simulink model "ClosedLoop"  (R2018b)
(part 3 of 12)

  "IW{1,1}(79,:)'" : Constant  Value=[0.15874800000000000022026824808563105762004852294921875;-0.25384499999999998731681216668221168220043182373046875;-0.29713800000000001322320031249546445906162261962890625]
      mask Display: e = 0.06;c1 = [120 150 230]/255;c2 = ([120 150 230]+0)/383;c3 = ([120 150 230]+128)/383;patch([0 1 1 0],[0 0 1 1],c1);patch([0 1 1 1-e 1-e 0+e],[0 0 1 1-e 0+e 0+e],c2);patch([0 0 1 1-e 0+e 0+e],[0 1 1 1-e 1-e 0+e],c3);plot([0 1 1 0 0],[0 0 1 1 0]);disp('Weights');
  "IW{1,1}(8,:)'" : Constant  Value=[-1.2600000000000000088817841970012523233890533447265625;-1.2874399999999999177902054725564084947109222412109375;0.01036259999999999958930629873066209256649017333984375]
      mask Display: e = 0.06;c1 = [120 150 230]/255;c2 = ([120 150 230]+0)/383;c3 = ([120 150 230]+128)/383;patch([0 1 1 0],[0 0 1 1],c1);patch([0 1 1 1-e 1-e 0+e],[0 0 1 1-e 0+e 0+e],c2);patch([0 0 1 1-e 0+e 0+e],[0 1 1 1-e 1-e 0+e],c3);plot([0 1 1 0 0],[0 0 1 1 0]);disp('Weights');
  "IW{1,1}(80,:)'" : Constant  Value=[0.048155099999999999293986974180370452813804149627685546875;0.0320770999999999972818187643497367389500141143798828125;-0.045470900000000001595079623939454904757440090179443359375]
      mask Display: e = 0.06;c1 = [120 150 230]/255;c2 = ([120 150 230]+0)/383;c3 = ([120 150 230]+128)/383;patch([0 1 1 0],[0 0 1 1],c1);patch([0 1 1 1-e 1-e 0+e],[0 0 1 1-e 0+e 0+e],c2);patch([0 0 1 1-e 0+e 0+e],[0 1 1 1-e 1-e 0+e],c3);plot([0 1 1 0 0],[0 0 1 1 0]);disp('Weights');
  "IW{1,1}(81,:)'" : Constant  Value=[0.007354610000000000140374378787555542658083140850067138671875;-0.0310646000000000012397638471384198055602610111236572265625;0.0233009999999999987962961967014052788726985454559326171875]
      mask Display: e = 0.06;c1 = [120 150 230]/255;c2 = ([120 150 230]+0)/383;c3 = ([120 150 230]+128)/383;patch([0 1 1 0],[0 0 1 1],c1);patch([0 1 1 1-e 1-e 0+e],[0 0 1 1-e 0+e 0+e],c2);patch([0 0 1 1-e 0+e 0+e],[0 1 1 1-e 1-e 0+e],c3);plot([0 1 1 0 0],[0 0 1 1 0]);disp('Weights');
  "IW{1,1}(82,:)'" : Constant  Value=[0.167198000000000013276491017677471973001956939697265625;-0.10580599999999999727418042994031566195189952850341796875;-0.1348669999999999868922628820655518211424350738525390625]
      mask Display: e = 0.06;c1 = [120 150 230]/255;c2 = ([120 150 230]+0)/383;c3 = ([120 150 230]+128)/383;patch([0 1 1 0],[0 0 1 1],c1);patch([0 1 1 1-e 1-e 0+e],[0 0 1 1-e 0+e 0+e],c2);patch([0 0 1 1-e 0+e 0+e],[0 1 1 1-e 1-e 0+e],c3);plot([0 1 1 0 0],[0 0 1 1 0]);disp('Weights');
  "IW{1,1}(83,:)'" : Constant  Value=[-0.00603968000000000039551029118456426658667623996734619140625;0.06340360000000000439968061982654035091400146484375;-0.090699899999999999966604491419275291264057159423828125]
      mask Display: e = 0.06;c1 = [120 150 230]/255;c2 = ([120 150 230]+0)/383;c3 = ([120 150 230]+128)/383;patch([0 1 1 0],[0 0 1 1],c1);patch([0 1 1 1-e 1-e 0+e],[0 0 1 1-e 0+e 0+e],c2);patch([0 0 1 1-e 0+e 0+e],[0 1 1 1-e 1-e 0+e],c3);plot([0 1 1 0 0],[0 0 1 1 0]);disp('Weights');
  "IW{1,1}(84,:)'" : Constant  Value=[0.1666640000000000065849548036567284725606441497802734375;-0.2229929999999999967741359796491451561450958251953125;-0.1958000000000000018207657603852567262947559356689453125]
      mask Display: e = 0.06;c1 = [120 150 230]/255;c2 = ([120 150 230]+0)/383;c3 = ([120 150 230]+128)/383;patch([0 1 1 0],[0 0 1 1],c1);patch([0 1 1 1-e 1-e 0+e],[0 0 1 1-e 0+e 0+e],c2);patch([0 0 1 1-e 0+e 0+e],[0 1 1 1-e 1-e 0+e],c3);plot([0 1 1 0 0],[0 0 1 1 0]);disp('Weights');
  "IW{1,1}(85,:)'" : Constant  Value=[-0.00359574000000000004728661906483466736972332000732421875;0.053989900000000000390709686826085089705884456634521484375;-0.057553399999999997616040303682893863879144191741943359375]
      mask Display: e = 0.06;c1 = [120 150 230]/255;c2 = ([120 150 230]+0)/383;c3 = ([120 150 230]+128)/383;patch([0 1 1 0],[0 0 1 1],c1);patch([0 1 1 1-e 1-e 0+e],[0 0 1 1-e 0+e 0+e],c2);patch([0 0 1 1-e 0+e 0+e],[0 1 1 1-e 1-e 0+e],c3);plot([0 1 1 0 0],[0 0 1 1 0]);disp('Weights');
  "IW{1,1}(86,:)'" : Constant  Value=[0.1475200000000000122302168392707244493067264556884765625;-0.147789000000000003698374939631321467459201812744140625;-0.2063450000000000006394884621840901672840118408203125]
      mask Display: e = 0.06;c1 = [120 150 230]/255;c2 = ([120 150 230]+0)/383;c3 = ([120 150 230]+128)/383;patch([0 1 1 0],[0 0 1 1],c1);patch([0 1 1 1-e 1-e 0+e],[0 0 1 1-e 0+e 0+e],c2);patch([0 0 1 1-e 0+e 0+e],[0 1 1 1-e 1-e 0+e],c3);plot([0 1 1 0 0],[0 0 1 1 0]);disp('Weights');
  "IW{1,1}(87,:)'" : Constant  Value=[-0.0066733399999999998275512780310236848890781402587890625;0.0222936000000000002219113781620762892998754978179931640625;-0.10869299999999999795097238575181108899414539337158203125]
      mask Display: e = 0.06;c1 = [120 150 230]/255;c2 = ([120 150 230]+0)/383;c3 = ([120 150 230]+128)/383;patch([0 1 1 0],[0 0 1 1],c1);patch([0 1 1 1-e 1-e 0+e],[0 0 1 1-e 0+e 0+e],c2);patch([0 0 1 1-e 0+e 0+e],[0 1 1 1-e 1-e 0+e],c3);plot([0 1 1 0 0],[0 0 1 1 0]);disp('Weights');
  "IW{1,1}(88,:)'" : Constant  Value=[0.055539600000000001467359567186576896347105503082275390625;0.01309800000000000026745272663220021058805286884307861328125;0.00212503999999999991510346575296352966688573360443115234375]
      mask Display: e = 0.06;c1 = [120 150 230]/255;c2 = ([120 150 230]+0)/383;c3 = ([120 150 230]+128)/383;patch([0 1 1 0],[0 0 1 1],c1);patch([0 1 1 1-e 1-e 0+e],[0 0 1 1-e 0+e 0+e],c2);patch([0 0 1 1-e 0+e 0+e],[0 1 1 1-e 1-e 0+e],c3);plot([0 1 1 0 0],[0 0 1 1 0]);disp('Weights');
  "IW{1,1}(89,:)'" : Constant  Value=[0.1697390000000000009894307595459395088255405426025390625;-0.164988999999999996770583265970344655215740203857421875;-0.1636229999999999906723502363092848099768161773681640625]
      mask Display: e = 0.06;c1 = [120 150 230]/255;c2 = ([120 150 230]+0)/383;c3 = ([120 150 230]+128)/383;patch([0 1 1 0],[0 0 1 1],c1);patch([0 1 1 1-e 1-e 0+e],[0 0 1 1-e 0+e 0+e],c2);patch([0 0 1 1-e 0+e 0+e],[0 1 1 1-e 1-e 0+e],c3);plot([0 1 1 0 0],[0 0 1 1 0]);disp('Weights');
  "IW{1,1}(9,:)'" : Constant  Value=[0.08682800000000000240074626844943850301206111907958984375;0.03627049999999999718713894480970338918268680572509765625;0.170582000000000011397105481592006981372833251953125]
      mask Display: e = 0.06;c1 = [120 150 230]/255;c2 = ([120 150 230]+0)/383;c3 = ([120 150 230]+128)/383;patch([0 1 1 0],[0 0 1 1],c1);patch([0 1 1 1-e 1-e 0+e],[0 0 1 1-e 0+e 0+e],c2);patch([0 0 1 1-e 0+e 0+e],[0 1 1 1-e 1-e 0+e],c3);plot([0 1 1 0 0],[0 0 1 1 0]);disp('Weights');
  "IW{1,1}(90,:)'" : Constant  Value=[-0.021500999999999999279243212413348373956978321075439453125;0.058919800000000001338751332013998762704432010650634765625;-0.09689589999999999314628240654201363213360309600830078125]
      mask Display: e = 0.06;c1 = [120 150 230]/255;c2 = ([120 150 230]+0)/383;c3 = ([120 150 230]+128)/383;patch([0 1 1 0],[0 0 1 1],c1);patch([0 1 1 1-e 1-e 0+e],[0 0 1 1-e 0+e 0+e],c2);patch([0 0 1 1-e 0+e 0+e],[0 1 1 1-e 1-e 0+e],c3);plot([0 1 1 0 0],[0 0 1 1 0]);disp('Weights');
  "IW{1,1}(91,:)'" : Constant  Value=[0.1663429999999999908677494886433123610913753509521484375;-0.28685199999999999587174670523381792008876800537109375;-0.30171300000000000895994389793486334383487701416015625]
      mask Display: e = 0.06;c1 = [120 150 230]/255;c2 = ([120 150 230]+0)/383;c3 = ([120 150 230]+128)/383;patch([0 1 1 0],[0 0 1 1],c1);patch([0 1 1 1-e 1-e 0+e],[0 0 1 1-e 0+e 0+e],c2);patch([0 0 1 1-e 0+e 0+e],[0 1 1 1-e 1-e 0+e],c3);plot([0 1 1 0 0],[0 0 1 1 0]);disp('Weights');
  "IW{1,1}(92,:)'" : Constant  Value=[0.11358699999999999352695567722548730671405792236328125;0.1527139999999999886437507257141987793147563934326171875;-0.074325699999999994549426673984271474182605743408203125]
      mask Display: e = 0.06;c1 = [120 150 230]/255;c2 = ([120 150 230]+0)/383;c3 = ([120 150 230]+128)/383;patch([0 1 1 0],[0 0 1 1],c1);patch([0 1 1 1-e 1-e 0+e],[0 0 1 1-e 0+e 0+e],c2);patch([0 0 1 1-e 0+e 0+e],[0 1 1 1-e 1-e 0+e],c3);plot([0 1 1 0 0],[0 0 1 1 0]);disp('Weights');
  "IW{1,1}(93,:)'" : Constant  Value=[0.015650799999999999434496800176930264569818973541259765625;-0.0078840500000000000857536264220470911823213100433349609375;-0.17593300000000000604671868131845258176326751708984375]
      mask Display: e = 0.06;c1 = [120 150 230]/255;c2 = ([120 150 230]+0)/383;c3 = ([120 150 230]+128)/383;patch([0 1 1 0],[0 0 1 1],c1);patch([0 1 1 1-e 1-e 0+e],[0 0 1 1-e 0+e 0+e],c2);patch([0 0 1 1-e 0+e 0+e],[0 1 1 1-e 1-e 0+e],c3);plot([0 1 1 0 0],[0 0 1 1 0]);disp('Weights');
  "IW{1,1}(94,:)'" : Constant  Value=[0.020723999999999999366284697543960646726191043853759765625;0.00929990999999999977398967843100763275288045406341552734375;0.08000590000000000479030148881065542809665203094482421875]
      mask Display: e = 0.06;c1 = [120 150 230]/255;c2 = ([120 150 230]+0)/383;c3 = ([120 150 230]+128)/383;patch([0 1 1 0],[0 0 1 1],c1);patch([0 1 1 1-e 1-e 0+e],[0 0 1 1-e 0+e 0+e],c2);patch([0 0 1 1-e 0+e 0+e],[0 1 1 1-e 1-e 0+e],c3);plot([0 1 1 0 0],[0 0 1 1 0]);disp('Weights');
  "IW{1,1}(95,:)'" : Constant  Value=[-0.0100663999999999996537436430799061781726777553558349609375;-0.01543590000000000066193717174201083253137767314910888671875;0.029199099999999998666933009872082038782536983489990234375]
      mask Display: e = 0.06;c1 = [120 150 230]/255;c2 = ([120 150 230]+0)/383;c3 = ([120 150 230]+128)/383;patch([0 1 1 0],[0 0 1 1],c1);patch([0 1 1 1-e 1-e 0+e],[0 0 1 1-e 0+e 0+e],c2);patch([0 0 1 1-e 0+e 0+e],[0 1 1 1-e 1-e 0+e],c3);plot([0 1 1 0 0],[0 0 1 1 0]);disp('Weights');
  "IW{1,1}(96,:)'" : Constant  Value=[0.0449270999999999975926812112447805702686309814453125;0.11766200000000000269739786062928033061325550079345703125;-0.081516599999999994619059862088761292397975921630859375]
      mask Display: e = 0.06;c1 = [120 150 230]/255;c2 = ([120 150 230]+0)/383;c3 = ([120 150 230]+128)/383;patch([0 1 1 0],[0 0 1 1],c1);patch([0 1 1 1-e 1-e 0+e],[0 0 1 1-e 0+e 0+e],c2);patch([0 0 1 1-e 0+e 0+e],[0 1 1 1-e 1-e 0+e],c3);plot([0 1 1 0 0],[0 0 1 1 0]);disp('Weights');
  "IW{1,1}(97,:)'" : Constant  Value=[0.00995095000000000007300826609935029409825801849365234375;-0.00017046199999999999525300553582241036565392278134822845458984375;0.047022500000000001796340853843503282405436038970947265625]
      mask Display: e = 0.06;c1 = [120 150 230]/255;c2 = ([120 150 230]+0)/383;c3 = ([120 150 230]+128)/383;patch([0 1 1 0],[0 0 1 1],c1);patch([0 1 1 1-e 1-e 0+e],[0 0 1 1-e 0+e 0+e],c2);patch([0 0 1 1-e 0+e 0+e],[0 1 1 1-e 1-e 0+e],c3);plot([0 1 1 0 0],[0 0 1 1 0]);disp('Weights');
  "IW{1,1}(98,:)'" : Constant  Value=[0.1802020000000000010675904604795505292713642120361328125;-0.1281940000000000023927526626721373759210109710693359375;-0.37388399999999999412381157526397146284580230712890625]
      mask Display: e = 0.06;c1 = [120 150 230]/255;c2 = ([120 150 230]+0)/383;c3 = ([120 150 230]+128)/383;patch([0 1 1 0],[0 0 1 1],c1);patch([0 1 1 1-e 1-e 0+e],[0 0 1 1-e 0+e 0+e],c2);patch([0 0 1 1-e 0+e 0+e],[0 1 1 1-e 1-e 0+e],c3);plot([0 1 1 0 0],[0 0 1 1 0]);disp('Weights');
  "IW{1,1}(99,:)'" : Constant  Value=[-0.016316299999999998859845362630949239246547222137451171875;-0.01379629999999999918902648943230815348215401172637939453125;0.07575020000000000364170915645445347763597965240478515625]
      mask Display: e = 0.06;c1 = [120 150 230]/255;c2 = ([120 150 230]+0)/383;c3 = ([120 150 230]+128)/383;patch([0 1 1 0],[0 0 1 1],c1);patch([0 1 1 1-e 1-e 0+e],[0 0 1 1-e 0+e 0+e],c2);patch([0 0 1 1-e 0+e 0+e],[0 1 1 1-e 1-e 0+e],c3);plot([0 1 1 0 0],[0 0 1 1 0]);disp('Weights');
  Mux : Mux  Inputs=300
      mask Display: e = 0.06;c1 = [120 150 230]/255;c2 = ([120 150 230]+0)/383;c3 = ([120 150 230]+128)/383;patch([0 1 1 0],[0 0 1 1],c1);patch([0 1 1 1-e 1-e 0+e],[0 0 1 1-e 0+e 0+e],c2);patch([0 0 1 1-e 0+e 0+e],[0 1 1 1-e 1-e 0+e],c3);plot([0 1 1 0 0],[0 0 1 1 0]);disp('Mux');
  dotprod{1..300} (300 alike) : neural/Weight Functions/dotprod
  "iz{1,1}" : Outport
      mask Display: e = 0.06;c1 = [120 230 180]/255;c2 = ([120 230 180]+0)/(256+128);c3 = ([120 230 180]+128)/(256+128);patch([0 1 1 0],[0 0 1 1],c1);patch([0 1 1 1-e 1-e 0+e],[0 0 1 1-e 0+e 0+e],c2);patch([0 0 1 1-e 0+e 0+e],[0 1 1 1-e 1-e 0+e],c3);plot([0 1 1 0 0],[0 0 1 1 0]);
  wires:
  Mux/1 -> "iz{1,1}"/1
  dotprod300/1 -> Mux/300
  "IW{1,1}(300,:)'"/1 -> dotprod300/1
  dotprod299/1 -> Mux/299
  "IW{1,1}(299,:)'"/1 -> dotprod299/1
  dotprod298/1 -> Mux/298
  "IW{1,1}(298,:)'"/1 -> dotprod298/1
  dotprod297/1 -> Mux/297
  "IW{1,1}(297,:)'"/1 -> dotprod297/1
  dotprod296/1 -> Mux/296
  "IW{1,1}(296,:)'"/1 -> dotprod296/1
  dotprod295/1 -> Mux/295
  "IW{1,1}(295,:)'"/1 -> dotprod295/1
  dotprod294/1 -> Mux/294
  "IW{1,1}(294,:)'"/1 -> dotprod294/1
  dotprod293/1 -> Mux/293
  "IW{1,1}(293,:)'"/1 -> dotprod293/1
  dotprod292/1 -> Mux/292
  "IW{1,1}(292,:)'"/1 -> dotprod292/1
  dotprod291/1 -> Mux/291
  "IW{1,1}(291,:)'"/1 -> dotprod291/1
  dotprod290/1 -> Mux/290
  "IW{1,1}(290,:)'"/1 -> dotprod290/1
  dotprod289/1 -> Mux/289
  "IW{1,1}(289,:)'"/1 -> dotprod289/1
  dotprod288/1 -> Mux/288
  "IW{1,1}(288,:)'"/1 -> dotprod288/1
  dotprod287/1 -> Mux/287
  "IW{1,1}(287,:)'"/1 -> dotprod287/1
  dotprod286/1 -> Mux/286
  "IW{1,1}(286,:)'"/1 -> dotprod286/1
  dotprod285/1 -> Mux/285
  "IW{1,1}(285,:)'"/1 -> dotprod285/1
  dotprod284/1 -> Mux/284
  "IW{1,1}(284,:)'"/1 -> dotprod284/1
  dotprod283/1 -> Mux/283
  "IW{1,1}(283,:)'"/1 -> dotprod283/1
  dotprod282/1 -> Mux/282
  "IW{1,1}(282,:)'"/1 -> dotprod282/1
  dotprod281/1 -> Mux/281
  "IW{1,1}(281,:)'"/1 -> dotprod281/1
  dotprod280/1 -> Mux/280
  "IW{1,1}(280,:)'"/1 -> dotprod280/1
  dotprod279/1 -> Mux/279
  "IW{1,1}(279,:)'"/1 -> dotprod279/1
  dotprod278/1 -> Mux/278
  "IW{1,1}(278,:)'"/1 -> dotprod278/1
  dotprod277/1 -> Mux/277
  "IW{1,1}(277,:)'"/1 -> dotprod277/1
  dotprod276/1 -> Mux/276
  "IW{1,1}(276,:)'"/1 -> dotprod276/1
  dotprod275/1 -> Mux/275
  "IW{1,1}(275,:)'"/1 -> dotprod275/1
  dotprod274/1 -> Mux/274
  "IW{1,1}(274,:)'"/1 -> dotprod274/1
  dotprod273/1 -> Mux/273
  "IW{1,1}(273,:)'"/1 -> dotprod273/1
  dotprod272/1 -> Mux/272
  "IW{1,1}(272,:)'"/1 -> dotprod272/1
  dotprod271/1 -> Mux/271
  "IW{1,1}(271,:)'"/1 -> dotprod271/1
  dotprod270/1 -> Mux/270
  "IW{1,1}(270,:)'"/1 -> dotprod270/1
  dotprod269/1 -> Mux/269
  "IW{1,1}(269,:)'"/1 -> dotprod269/1
  dotprod268/1 -> Mux/268
  "IW{1,1}(268,:)'"/1 -> dotprod268/1
  dotprod267/1 -> Mux/267
  "IW{1,1}(267,:)'"/1 -> dotprod267/1
  dotprod266/1 -> Mux/266
  "IW{1,1}(266,:)'"/1 -> dotprod266/1
  dotprod265/1 -> Mux/265
  "IW{1,1}(265,:)'"/1 -> dotprod265/1
  dotprod264/1 -> Mux/264
  "IW{1,1}(264,:)'"/1 -> dotprod264/1
  dotprod263/1 -> Mux/263
  "IW{1,1}(263,:)'"/1 -> dotprod263/1
  dotprod262/1 -> Mux/262
  "IW{1,1}(262,:)'"/1 -> dotprod262/1
  dotprod261/1 -> Mux/261
  "IW{1,1}(261,:)'"/1 -> dotprod261/1
  dotprod260/1 -> Mux/260
  "IW{1,1}(260,:)'"/1 -> dotprod260/1
  dotprod259/1 -> Mux/259
  "IW{1,1}(259,:)'"/1 -> dotprod259/1
  dotprod258/1 -> Mux/258
  "IW{1,1}(258,:)'"/1 -> dotprod258/1
  dotprod257/1 -> Mux/257
  "IW{1,1}(257,:)'"/1 -> dotprod257/1
  dotprod256/1 -> Mux/256
  "IW{1,1}(256,:)'"/1 -> dotprod256/1
  dotprod255/1 -> Mux/255
  "IW{1,1}(255,:)'"/1 -> dotprod255/1
  dotprod254/1 -> Mux/254
  "IW{1,1}(254,:)'"/1 -> dotprod254/1
  dotprod253/1 -> Mux/253
  "IW{1,1}(253,:)'"/1 -> dotprod253/1
  dotprod252/1 -> Mux/252
  "IW{1,1}(252,:)'"/1 -> dotprod252/1
  dotprod251/1 -> Mux/251
  "IW{1,1}(251,:)'"/1 -> dotprod251/1
  dotprod250/1 -> Mux/250
  "IW{1,1}(250,:)'"/1 -> dotprod250/1
  dotprod249/1 -> Mux/249
  "IW{1,1}(249,:)'"/1 -> dotprod249/1
  dotprod248/1 -> Mux/248
  "IW{1,1}(248,:)'"/1 -> dotprod248/1
  dotprod247/1 -> Mux/247
  "IW{1,1}(247,:)'"/1 -> dotprod247/1
  dotprod246/1 -> Mux/246
  "IW{1,1}(246,:)'"/1 -> dotprod246/1
  dotprod245/1 -> Mux/245
  "IW{1,1}(245,:)'"/1 -> dotprod245/1
  dotprod244/1 -> Mux/244
  "IW{1,1}(244,:)'"/1 -> dotprod244/1
  dotprod243/1 -> Mux/243
  "IW{1,1}(243,:)'"/1 -> dotprod243/1
  dotprod242/1 -> Mux/242
  "IW{1,1}(242,:)'"/1 -> dotprod242/1
  dotprod241/1 -> Mux/241
  "IW{1,1}(241,:)'"/1 -> dotprod241/1
  dotprod240/1 -> Mux/240
  "IW{1,1}(240,:)'"/1 -> dotprod240/1
  dotprod239/1 -> Mux/239
  "IW{1,1}(239,:)'"/1 -> dotprod239/1
  dotprod238/1 -> Mux/238
  "IW{1,1}(238,:)'"/1 -> dotprod238/1
  dotprod237/1 -> Mux/237
  "IW{1,1}(237,:)'"/1 -> dotprod237/1
  dotprod236/1 -> Mux/236
  "IW{1,1}(236,:)'"/1 -> dotprod236/1
  dotprod235/1 -> Mux/235
  "IW{1,1}(235,:)'"/1 -> dotprod235/1
  dotprod234/1 -> Mux/234
  "IW{1,1}(234,:)'"/1 -> dotprod234/1
  dotprod233/1 -> Mux/233
  "IW{1,1}(233,:)'"/1 -> dotprod233/1
  dotprod232/1 -> Mux/232
  "IW{1,1}(232,:)'"/1 -> dotprod232/1
  dotprod231/1 -> Mux/231
  "IW{1,1}(231,:)'"/1 -> dotprod231/1
  dotprod230/1 -> Mux/230
  "IW{1,1}(230,:)'"/1 -> dotprod230/1
  dotprod229/1 -> Mux/229
  "IW{1,1}(229,:)'"/1 -> dotprod229/1
  dotprod228/1 -> Mux/228
  "IW{1,1}(228,:)'"/1 -> dotprod228/1
  dotprod227/1 -> Mux/227
  "IW{1,1}(227,:)'"/1 -> dotprod227/1
  dotprod226/1 -> Mux/226
  "IW{1,1}(226,:)'"/1 -> dotprod226/1
  dotprod225/1 -> Mux/225
  "IW{1,1}(225,:)'"/1 -> dotprod225/1
  dotprod224/1 -> Mux/224
  "IW{1,1}(224,:)'"/1 -> dotprod224/1
  dotprod223/1 -> Mux/223
  "IW{1,1}(223,:)'"/1 -> dotprod223/1
  dotprod222/1 -> Mux/222
  "IW{1,1}(222,:)'"/1 -> dotprod222/1
  dotprod221/1 -> Mux/221
  "IW{1,1}(221,:)'"/1 -> dotprod221/1
  dotprod220/1 -> Mux/220
  "IW{1,1}(220,:)'"/1 -> dotprod220/1
  dotprod219/1 -> Mux/219
  "IW{1,1}(219,:)'"/1 -> dotprod219/1
  dotprod218/1 -> Mux/218
  "IW{1,1}(218,:)'"/1 -> dotprod218/1
  dotprod217/1 -> Mux/217
  "IW{1,1}(217,:)'"/1 -> dotprod217/1
  dotprod216/1 -> Mux/216
  "IW{1,1}(216,:)'"/1 -> dotprod216/1
  dotprod215/1 -> Mux/215
  "IW{1,1}(215,:)'"/1 -> dotprod215/1
  dotprod214/1 -> Mux/214
  "IW{1,1}(214,:)'"/1 -> dotprod214/1
  dotprod213/1 -> Mux/213
  "IW{1,1}(213,:)'"/1 -> dotprod213/1
  dotprod212/1 -> Mux/212
  "IW{1,1}(212,:)'"/1 -> dotprod212/1
  dotprod211/1 -> Mux/211
  "IW{1,1}(211,:)'"/1 -> dotprod211/1
  dotprod210/1 -> Mux/210
  "IW{1,1}(210,:)'"/1 -> dotprod210/1
  dotprod209/1 -> Mux/209
  "IW{1,1}(209,:)'"/1 -> dotprod209/1
  dotprod208/1 -> Mux/208
  "IW{1,1}(208,:)'"/1 -> dotprod208/1
  dotprod207/1 -> Mux/207
  "IW{1,1}(207,:)'"/1 -> dotprod207/1
  dotprod206/1 -> Mux/206
  "IW{1,1}(206,:)'"/1 -> dotprod206/1
  dotprod205/1 -> Mux/205
  "IW{1,1}(205,:)'"/1 -> dotprod205/1
  dotprod204/1 -> Mux/204
  "IW{1,1}(204,:)'"/1 -> dotprod204/1
  dotprod203/1 -> Mux/203
  "IW{1,1}(203,:)'"/1 -> dotprod203/1
  dotprod202/1 -> Mux/202
  "IW{1,1}(202,:)'"/1 -> dotprod202/1
  dotprod201/1 -> Mux/201
  "IW{1,1}(201,:)'"/1 -> dotprod201/1
  dotprod200/1 -> Mux/200
  "IW{1,1}(200,:)'"/1 -> dotprod200/1
  dotprod199/1 -> Mux/199
  "IW{1,1}(199,:)'"/1 -> dotprod199/1
  dotprod198/1 -> Mux/198
  "IW{1,1}(198,:)'"/1 -> dotprod198/1
  dotprod197/1 -> Mux/197
  "IW{1,1}(197,:)'"/1 -> dotprod197/1
  dotprod196/1 -> Mux/196
  "IW{1,1}(196,:)'"/1 -> dotprod196/1
  dotprod195/1 -> Mux/195
  "IW{1,1}(195,:)'"/1 -> dotprod195/1
  dotprod194/1 -> Mux/194
  "IW{1,1}(194,:)'"/1 -> dotprod194/1
  dotprod193/1 -> Mux/193
  "IW{1,1}(193,:)'"/1 -> dotprod193/1
  dotprod192/1 -> Mux/192
  "IW{1,1}(192,:)'"/1 -> dotprod192/1
  dotprod191/1 -> Mux/191
  "IW{1,1}(191,:)'"/1 -> dotprod191/1
  dotprod190/1 -> Mux/190
  "IW{1,1}(190,:)'"/1 -> dotprod190/1
  dotprod189/1 -> Mux/189
  "IW{1,1}(189,:)'"/1 -> dotprod189/1
  dotprod188/1 -> Mux/188
  "IW{1,1}(188,:)'"/1 -> dotprod188/1
  dotprod187/1 -> Mux/187
  "IW{1,1}(187,:)'"/1 -> dotprod187/1
  dotprod186/1 -> Mux/186
  "IW{1,1}(186,:)'"/1 -> dotprod186/1
  dotprod185/1 -> Mux/185
  "IW{1,1}(185,:)'"/1 -> dotprod185/1
  dotprod184/1 -> Mux/184
  "IW{1,1}(184,:)'"/1 -> dotprod184/1
  dotprod183/1 -> Mux/183
  "IW{1,1}(183,:)'"/1 -> dotprod183/1
  dotprod182/1 -> Mux/182
  "IW{1,1}(182,:)'"/1 -> dotprod182/1
  dotprod181/1 -> Mux/181
  "IW{1,1}(181,:)'"/1 -> dotprod181/1
  dotprod180/1 -> Mux/180
  "IW{1,1}(180,:)'"/1 -> dotprod180/1
  dotprod179/1 -> Mux/179
  "IW{1,1}(179,:)'"/1 -> dotprod179/1
  dotprod178/1 -> Mux/178
  "IW{1,1}(178,:)'"/1 -> dotprod178/1
  dotprod177/1 -> Mux/177
  "IW{1,1}(177,:)'"/1 -> dotprod177/1
  dotprod176/1 -> Mux/176
  "IW{1,1}(176,:)'"/1 -> dotprod176/1
  dotprod175/1 -> Mux/175
  "IW{1,1}(175,:)'"/1 -> dotprod175/1
  dotprod174/1 -> Mux/174
  "IW{1,1}(174,:)'"/1 -> dotprod174/1
  dotprod173/1 -> Mux/173
  "IW{1,1}(173,:)'"/1 -> dotprod173/1
  dotprod172/1 -> Mux/172
  "IW{1,1}(172,:)'"/1 -> dotprod172/1
  dotprod171/1 -> Mux/171
  "IW{1,1}(171,:)'"/1 -> dotprod171/1
  dotprod170/1 -> Mux/170
  "IW{1,1}(170,:)'"/1 -> dotprod170/1
  dotprod169/1 -> Mux/169
  "IW{1,1}(169,:)'"/1 -> dotprod169/1
  dotprod168/1 -> Mux/168
  "IW{1,1}(168,:)'"/1 -> dotprod168/1
  dotprod167/1 -> Mux/167
  "IW{1,1}(167,:)'"/1 -> dotprod167/1
  dotprod166/1 -> Mux/166
  "IW{1,1}(166,:)'"/1 -> dotprod166/1
  dotprod165/1 -> Mux/165
  "IW{1,1}(165,:)'"/1 -> dotprod165/1
  dotprod164/1 -> Mux/164
  "IW{1,1}(164,:)'"/1 -> dotprod164/1
  dotprod163/1 -> Mux/163
  "IW{1,1}(163,:)'"/1 -> dotprod163/1
  dotprod162/1 -> Mux/162
  "IW{1,1}(162,:)'"/1 -> dotprod162/1
  dotprod161/1 -> Mux/161
  "IW{1,1}(161,:)'"/1 -> dotprod161/1
  dotprod160/1 -> Mux/160
  "IW{1,1}(160,:)'"/1 -> dotprod160/1
  dotprod159/1 -> Mux/159
  "IW{1,1}(159,:)'"/1 -> dotprod159/1
  dotprod158/1 -> Mux/158
  "IW{1,1}(158,:)'"/1 -> dotprod158/1
  dotprod157/1 -> Mux/157
  "IW{1,1}(157,:)'"/1 -> dotprod157/1
  dotprod156/1 -> Mux/156
  "IW{1,1}(156,:)'"/1 -> dotprod156/1
  dotprod155/1 -> Mux/155
  "IW{1,1}(155,:)'"/1 -> dotprod155/1
  dotprod154/1 -> Mux/154
  "IW{1,1}(154,:)'"/1 -> dotprod154/1
  dotprod153/1 -> Mux/153
  "IW{1,1}(153,:)'"/1 -> dotprod153/1
  dotprod152/1 -> Mux/152
  "IW{1,1}(152,:)'"/1 -> dotprod152/1
  dotprod151/1 -> Mux/151
  "IW{1,1}(151,:)'"/1 -> dotprod151/1
  dotprod150/1 -> Mux/150
  "IW{1,1}(150,:)'"/1 -> dotprod150/1
  dotprod149/1 -> Mux/149
  "IW{1,1}(149,:)'"/1 -> dotprod149/1
  dotprod148/1 -> Mux/148
  "IW{1,1}(148,:)'"/1 -> dotprod148/1
  dotprod147/1 -> Mux/147
  "IW{1,1}(147,:)'"/1 -> dotprod147/1
  dotprod146/1 -> Mux/146
  "IW{1,1}(146,:)'"/1 -> dotprod146/1
  dotprod145/1 -> Mux/145
  "IW{1,1}(145,:)'"/1 -> dotprod145/1
  dotprod144/1 -> Mux/144
  "IW{1,1}(144,:)'"/1 -> dotprod144/1
  dotprod143/1 -> Mux/143
  "IW{1,1}(143,:)'"/1 -> dotprod143/1
  dotprod142/1 -> Mux/142
  "IW{1,1}(142,:)'"/1 -> dotprod142/1
  dotprod141/1 -> Mux/141
  "IW{1,1}(141,:)'"/1 -> dotprod141/1
  dotprod140/1 -> Mux/140
  "IW{1,1}(140,:)'"/1 -> dotprod140/1
  dotprod139/1 -> Mux/139
  "IW{1,1}(139,:)'"/1 -> dotprod139/1
  dotprod138/1 -> Mux/138
  "IW{1,1}(138,:)'"/1 -> dotprod138/1
  dotprod137/1 -> Mux/137
  "IW{1,1}(137,:)'"/1 -> dotprod137/1
  dotprod136/1 -> Mux/136
  "IW{1,1}(136,:)'"/1 -> dotprod136/1
  dotprod135/1 -> Mux/135
  "IW{1,1}(135,:)'"/1 -> dotprod135/1
  dotprod134/1 -> Mux/134
  "IW{1,1}(134,:)'"/1 -> dotprod134/1
  dotprod133/1 -> Mux/133
  "IW{1,1}(133,:)'"/1 -> dotprod133/1
  dotprod132/1 -> Mux/132
  "IW{1,1}(132,:)'"/1 -> dotprod132/1
  dotprod131/1 -> Mux/131
  "IW{1,1}(131,:)'"/1 -> dotprod131/1
  dotprod130/1 -> Mux/130
  "IW{1,1}(130,:)'"/1 -> dotprod130/1
  dotprod129/1 -> Mux/129
  "IW{1,1}(129,:)'"/1 -> dotprod129/1
  dotprod128/1 -> Mux/128
  "IW{1,1}(128,:)'"/1 -> dotprod128/1
  dotprod127/1 -> Mux/127
  "IW{1,1}(127,:)'"/1 -> dotprod127/1
  dotprod126/1 -> Mux/126
  "IW{1,1}(126,:)'"/1 -> dotprod126/1
  dotprod125/1 -> Mux/125
  "IW{1,1}(125,:)'"/1 -> dotprod125/1
  dotprod124/1 -> Mux/124
  "IW{1,1}(124,:)'"/1 -> dotprod124/1
  dotprod123/1 -> Mux/123
  "IW{1,1}(123,:)'"/1 -> dotprod123/1
  dotprod122/1 -> Mux/122
  "IW{1,1}(122,:)'"/1 -> dotprod122/1
  dotprod121/1 -> Mux/121
  "IW{1,1}(121,:)'"/1 -> dotprod121/1
  dotprod120/1 -> Mux/120
  "IW{1,1}(120,:)'"/1 -> dotprod120/1
  dotprod119/1 -> Mux/119
  "IW{1,1}(119,:)'"/1 -> dotprod119/1
  dotprod118/1 -> Mux/118
  "IW{1,1}(118,:)'"/1 -> dotprod118/1
  dotprod117/1 -> Mux/117
  "IW{1,1}(117,:)'"/1 -> dotprod117/1
  dotprod116/1 -> Mux/116
  "IW{1,1}(116,:)'"/1 -> dotprod116/1
  dotprod115/1 -> Mux/115
  "IW{1,1}(115,:)'"/1 -> dotprod115/1
  dotprod114/1 -> Mux/114
  "IW{1,1}(114,:)'"/1 -> dotprod114/1
  dotprod113/1 -> Mux/113
  "IW{1,1}(113,:)'"/1 -> dotprod113/1
  dotprod112/1 -> Mux/112
  "IW{1,1}(112,:)'"/1 -> dotprod112/1
  dotprod111/1 -> Mux/111
  "IW{1,1}(111,:)'"/1 -> dotprod111/1
  dotprod110/1 -> Mux/110
  "IW{1,1}(110,:)'"/1 -> dotprod110/1
  dotprod109/1 -> Mux/109
  "IW{1,1}(109,:)'"/1 -> dotprod109/1
  dotprod108/1 -> Mux/108
  "IW{1,1}(108,:)'"/1 -> dotprod108/1
  dotprod107/1 -> Mux/107
  "IW{1,1}(107,:)'"/1 -> dotprod107/1
  dotprod106/1 -> Mux/106
  "IW{1,1}(106,:)'"/1 -> dotprod106/1
  dotprod105/1 -> Mux/105
  "IW{1,1}(105,:)'"/1 -> dotprod105/1
  dotprod104/1 -> Mux/104
  "IW{1,1}(104,:)'"/1 -> dotprod104/1
  dotprod103/1 -> Mux/103
  "IW{1,1}(103,:)'"/1 -> dotprod103/1
  dotprod102/1 -> Mux/102
  "IW{1,1}(102,:)'"/1 -> dotprod102/1
  dotprod101/1 -> Mux/101
  "IW{1,1}(101,:)'"/1 -> dotprod101/1
  dotprod100/1 -> Mux/100
  "IW{1,1}(100,:)'"/1 -> dotprod100/1
  dotprod99/1 -> Mux/99
  "IW{1,1}(99,:)'"/1 -> dotprod99/1
  dotprod98/1 -> Mux/98
  "IW{1,1}(98,:)'"/1 -> dotprod98/1
  dotprod97/1 -> Mux/97
  "IW{1,1}(97,:)'"/1 -> dotprod97/1
  dotprod96/1 -> Mux/96
  "IW{1,1}(96,:)'"/1 -> dotprod96/1
  dotprod95/1 -> Mux/95
  "IW{1,1}(95,:)'"/1 -> dotprod95/1
  dotprod94/1 -> Mux/94
  "IW{1,1}(94,:)'"/1 -> dotprod94/1
  dotprod93/1 -> Mux/93
  "IW{1,1}(93,:)'"/1 -> dotprod93/1
  dotprod92/1 -> Mux/92
  "IW{1,1}(92,:)'"/1 -> dotprod92/1
  dotprod91/1 -> Mux/91
  "IW{1,1}(91,:)'"/1 -> dotprod91/1
  dotprod90/1 -> Mux/90
  "IW{1,1}(90,:)'"/1 -> dotprod90/1
  dotprod89/1 -> Mux/89
  "IW{1,1}(89,:)'"/1 -> dotprod89/1
  dotprod88/1 -> Mux/88
  "IW{1,1}(88,:)'"/1 -> dotprod88/1
  dotprod87/1 -> Mux/87
  "IW{1,1}(87,:)'"/1 -> dotprod87/1
  dotprod86/1 -> Mux/86
  "IW{1,1}(86,:)'"/1 -> dotprod86/1
  dotprod85/1 -> Mux/85
  "IW{1,1}(85,:)'"/1 -> dotprod85/1
  dotprod84/1 -> Mux/84
  "IW{1,1}(84,:)'"/1 -> dotprod84/1
  dotprod83/1 -> Mux/83
  "IW{1,1}(83,:)'"/1 -> dotprod83/1
  dotprod82/1 -> Mux/82
  "IW{1,1}(82,:)'"/1 -> dotprod82/1
  dotprod81/1 -> Mux/81
  "IW{1,1}(81,:)'"/1 -> dotprod81/1
  dotprod80/1 -> Mux/80
  "IW{1,1}(80,:)'"/1 -> dotprod80/1
  dotprod79/1 -> Mux/79
  "IW{1,1}(79,:)'"/1 -> dotprod79/1
  dotprod78/1 -> Mux/78
  "IW{1,1}(78,:)'"/1 -> dotprod78/1
  dotprod77/1 -> Mux/77
  "IW{1,1}(77,:)'"/1 -> dotprod77/1
  dotprod76/1 -> Mux/76
  "IW{1,1}(76,:)'"/1 -> dotprod76/1
  dotprod75/1 -> Mux/75
  "IW{1,1}(75,:)'"/1 -> dotprod75/1
  dotprod74/1 -> Mux/74
  "IW{1,1}(74,:)'"/1 -> dotprod74/1
  dotprod73/1 -> Mux/73
  "IW{1,1}(73,:)'"/1 -> dotprod73/1
  dotprod72/1 -> Mux/72
  "IW{1,1}(72,:)'"/1 -> dotprod72/1
  dotprod71/1 -> Mux/71
  "IW{1,1}(71,:)'"/1 -> dotprod71/1
  dotprod70/1 -> Mux/70
  "IW{1,1}(70,:)'"/1 -> dotprod70/1
  dotprod69/1 -> Mux/69
  "IW{1,1}(69,:)'"/1 -> dotprod69/1
  dotprod68/1 -> Mux/68
  "IW{1,1}(68,:)'"/1 -> dotprod68/1
  dotprod67/1 -> Mux/67
  "IW{1,1}(67,:)'"/1 -> dotprod67/1
  dotprod66/1 -> Mux/66
  "IW{1,1}(66,:)'"/1 -> dotprod66/1
  dotprod65/1 -> Mux/65
  "IW{1,1}(65,:)'"/1 -> dotprod65/1
  dotprod64/1 -> Mux/64
  "IW{1,1}(64,:)'"/1 -> dotprod64/1
  dotprod63/1 -> Mux/63
  "IW{1,1}(63,:)'"/1 -> dotprod63/1
  dotprod62/1 -> Mux/62
  "IW{1,1}(62,:)'"/1 -> dotprod62/1
  dotprod61/1 -> Mux/61
  "IW{1,1}(61,:)'"/1 -> dotprod61/1
  dotprod60/1 -> Mux/60
  "IW{1,1}(60,:)'"/1 -> dotprod60/1
  dotprod59/1 -> Mux/59
  "IW{1,1}(59,:)'"/1 -> dotprod59/1
  dotprod58/1 -> Mux/58
  "IW{1,1}(58,:)'"/1 -> dotprod58/1
  dotprod57/1 -> Mux/57
  "IW{1,1}(57,:)'"/1 -> dotprod57/1
  dotprod56/1 -> Mux/56
  "IW{1,1}(56,:)'"/1 -> dotprod56/1
  dotprod55/1 -> Mux/55
  "IW{1,1}(55,:)'"/1 -> dotprod55/1
  dotprod54/1 -> Mux/54
  "IW{1,1}(54,:)'"/1 -> dotprod54/1
  dotprod53/1 -> Mux/53
  "IW{1,1}(53,:)'"/1 -> dotprod53/1
  dotprod52/1 -> Mux/52
  "IW{1,1}(52,:)'"/1 -> dotprod52/1
  dotprod51/1 -> Mux/51
  "IW{1,1}(51,:)'"/1 -> dotprod51/1
  dotprod50/1 -> Mux/50
  "IW{1,1}(50,:)'"/1 -> dotprod50/1
  dotprod49/1 -> Mux/49
  "IW{1,1}(49,:)'"/1 -> dotprod49/1
  dotprod48/1 -> Mux/48
  "IW{1,1}(48,:)'"/1 -> dotprod48/1
  dotprod47/1 -> Mux/47
  "IW{1,1}(47,:)'"/1 -> dotprod47/1
  dotprod46/1 -> Mux/46
  "IW{1,1}(46,:)'"/1 -> dotprod46/1
  dotprod45/1 -> Mux/45
  "IW{1,1}(45,:)'"/1 -> dotprod45/1
  dotprod44/1 -> Mux/44
  "IW{1,1}(44,:)'"/1 -> dotprod44/1
  dotprod43/1 -> Mux/43
  "IW{1,1}(43,:)'"/1 -> dotprod43/1
  dotprod42/1 -> Mux/42
  "IW{1,1}(42,:)'"/1 -> dotprod42/1
  dotprod41/1 -> Mux/41
  "IW{1,1}(41,:)'"/1 -> dotprod41/1
  dotprod40/1 -> Mux/40
  "IW{1,1}(40,:)'"/1 -> dotprod40/1
  dotprod39/1 -> Mux/39
  "IW{1,1}(39,:)'"/1 -> dotprod39/1
  dotprod38/1 -> Mux/38
  "IW{1,1}(38,:)'"/1 -> dotprod38/1
  dotprod37/1 -> Mux/37
  "IW{1,1}(37,:)'"/1 -> dotprod37/1
  dotprod36/1 -> Mux/36
  "IW{1,1}(36,:)'"/1 -> dotprod36/1
  dotprod35/1 -> Mux/35
  "IW{1,1}(35,:)'"/1 -> dotprod35/1
  dotprod34/1 -> Mux/34
  "IW{1,1}(34,:)'"/1 -> dotprod34/1
  dotprod33/1 -> Mux/33
  "IW{1,1}(33,:)'"/1 -> dotprod33/1
  dotprod32/1 -> Mux/32
  "IW{1,1}(32,:)'"/1 -> dotprod32/1
  dotprod31/1 -> Mux/31
  "IW{1,1}(31,:)'"/1 -> dotprod31/1
  dotprod30/1 -> Mux/30
  "IW{1,1}(30,:)'"/1 -> dotprod30/1
  dotprod29/1 -> Mux/29
  "IW{1,1}(29,:)'"/1 -> dotprod29/1
  dotprod28/1 -> Mux/28
  "IW{1,1}(28,:)'"/1 -> dotprod28/1
  dotprod27/1 -> Mux/27
  "IW{1,1}(27,:)'"/1 -> dotprod27/1
  dotprod26/1 -> Mux/26
  "IW{1,1}(26,:)'"/1 -> dotprod26/1
  dotprod25/1 -> Mux/25
  "IW{1,1}(25,:)'"/1 -> dotprod25/1
  dotprod24/1 -> Mux/24
  "IW{1,1}(24,:)'"/1 -> dotprod24/1
  dotprod23/1 -> Mux/23
  "IW{1,1}(23,:)'"/1 -> dotprod23/1
  dotprod22/1 -> Mux/22
  "IW{1,1}(22,:)'"/1 -> dotprod22/1
  dotprod21/1 -> Mux/21
  "IW{1,1}(21,:)'"/1 -> dotprod21/1
  dotprod20/1 -> Mux/20
  "IW{1,1}(20,:)'"/1 -> dotprod20/1
  dotprod19/1 -> Mux/19
  "IW{1,1}(19,:)'"/1 -> dotprod19/1
  dotprod18/1 -> Mux/18
  "IW{1,1}(18,:)'"/1 -> dotprod18/1
  dotprod17/1 -> Mux/17
  "IW{1,1}(17,:)'"/1 -> dotprod17/1
  dotprod16/1 -> Mux/16
  "IW{1,1}(16,:)'"/1 -> dotprod16/1
  dotprod15/1 -> Mux/15
  "IW{1,1}(15,:)'"/1 -> dotprod15/1
  dotprod14/1 -> Mux/14
  "IW{1,1}(14,:)'"/1 -> dotprod14/1
  dotprod13/1 -> Mux/13
  "IW{1,1}(13,:)'"/1 -> dotprod13/1
  dotprod12/1 -> Mux/12
  "IW{1,1}(12,:)'"/1 -> dotprod12/1
  dotprod11/1 -> Mux/11
  "IW{1,1}(11,:)'"/1 -> dotprod11/1
  dotprod10/1 -> Mux/10
  "IW{1,1}(10,:)'"/1 -> dotprod10/1
  dotprod9/1 -> Mux/9
  "IW{1,1}(9,:)'"/1 -> dotprod9/1
  dotprod8/1 -> Mux/8
  "IW{1,1}(8,:)'"/1 -> dotprod8/1
  dotprod7/1 -> Mux/7
  "IW{1,1}(7,:)'"/1 -> dotprod7/1
  dotprod6/1 -> Mux/6
  "IW{1,1}(6,:)'"/1 -> dotprod6/1
  dotprod5/1 -> Mux/5
  "IW{1,1}(5,:)'"/1 -> dotprod5/1
  dotprod4/1 -> Mux/4
  "IW{1,1}(4,:)'"/1 -> dotprod4/1
  dotprod3/1 -> Mux/3
  "IW{1,1}(3,:)'"/1 -> dotprod3/1
  dotprod2/1 -> Mux/2
  "IW{1,1}(2,:)'"/1 -> dotprod2/1
  dotprod1/1 -> Mux/1
  "pd{1,1}"/1 -> dotprod300/2, dotprod299/2, dotprod298/2, dotprod297/2, dotprod296/2, dotprod295/2, dotprod294/2, dotprod293/2, dotprod292/2, dotprod291/2, dotprod290/2, dotprod289/2, dotprod288/2, dotprod287/2, dotprod286/2, dotprod285/2, dotprod284/2, dotprod283/2, dotprod282/2, dotprod281/2, dotprod280/2, dotprod279/2, dotprod278/2, dotprod277/2, dotprod276/2, dotprod275/2, dotprod274/2, dotprod273/2, dotprod272/2, dotprod271/2, dotprod270/2, dotprod269/2, dotprod268/2, dotprod267/2, dotprod266/2, dotprod265/2, dotprod264/2, dotprod263/2, dotprod262/2, dotprod261/2, dotprod260/2, dotprod259/2, dotprod258/2, dotprod257/2, dotprod256/2, dotprod255/2, dotprod254/2, dotprod253/2, dotprod252/2, dotprod251/2, dotprod250/2, dotprod249/2, dotprod248/2, dotprod247/2, dotprod246/2, dotprod245/2, dotprod244/2, dotprod243/2, dotprod242/2, dotprod241/2, dotprod240/2, dotprod239/2, dotprod238/2, dotprod237/2, dotprod236/2, dotprod235/2, dotprod234/2, dotprod233/2, dotprod232/2, dotprod231/2, dotprod230/2, dotprod229/2, dotprod228/2, dotprod227/2, dotprod226/2, dotprod225/2, dotprod224/2, dotprod223/2, dotprod222/2, dotprod221/2, dotprod220/2, dotprod219/2, dotprod218/2, dotprod217/2, dotprod216/2, dotprod215/2, dotprod214/2, dotprod213/2, dotprod212/2, dotprod211/2, dotprod210/2, dotprod209/2, dotprod208/2, dotprod207/2, dotprod206/2, dotprod205/2, dotprod204/2, dotprod203/2, dotprod202/2, dotprod201/2, dotprod200/2, dotprod199/2, dotprod198/2, dotprod197/2, dotprod196/2, dotprod195/2, dotprod194/2, dotprod193/2, dotprod192/2, dotprod191/2, dotprod190/2, dotprod189/2, dotprod188/2, dotprod187/2, dotprod186/2, dotprod185/2, dotprod184/2, dotprod183/2, dotprod182/2, dotprod181/2, dotprod180/2, dotprod179/2, dotprod178/2, dotprod177/2, dotprod176/2, dotprod175/2, dotprod174/2, dotprod173/2, dotprod172/2, dotprod171/2, dotprod170/2, dotprod169/2, dotprod168/2, dotprod167/2, dotprod166/2, dotprod165/2, dotprod164/2, dotprod163/2, dotprod162/2, dotprod161/2, dotprod160/2, dotprod159/2, dotprod158/2, dotprod157/2, dotprod156/2, dotprod155/2, dotprod154/2, dotprod153/2, dotprod152/2, dotprod151/2, dotprod150/2, dotprod149/2, dotprod148/2, dotprod147/2, dotprod146/2, dotprod145/2, dotprod144/2, dotprod143/2, dotprod142/2, dotprod141/2, dotprod140/2, dotprod139/2, dotprod138/2, dotprod137/2, dotprod136/2, dotprod135/2, dotprod134/2, dotprod133/2, dotprod132/2, dotprod131/2, dotprod130/2, dotprod129/2, dotprod128/2, dotprod127/2, dotprod126/2, dotprod125/2, dotprod124/2, dotprod123/2, dotprod122/2, dotprod121/2, dotprod120/2, dotprod119/2, dotprod118/2, dotprod117/2, dotprod116/2, dotprod115/2, dotprod114/2, dotprod113/2, dotprod112/2, dotprod111/2, dotprod110/2, dotprod109/2, dotprod108/2, dotprod107/2, dotprod106/2, dotprod105/2, dotprod104/2, dotprod103/2, dotprod102/2, dotprod101/2, dotprod100/2, dotprod99/2, dotprod98/2, dotprod97/2, dotprod96/2, dotprod95/2, dotprod94/2, dotprod93/2, dotprod92/2, dotprod91/2, dotprod90/2, dotprod89/2, dotprod88/2, dotprod87/2, dotprod86/2, dotprod85/2, dotprod84/2, dotprod83/2, dotprod82/2, dotprod81/2, dotprod80/2, dotprod79/2, dotprod78/2, dotprod77/2, dotprod76/2, dotprod75/2, dotprod74/2, dotprod73/2, dotprod72/2, dotprod71/2, dotprod70/2, dotprod69/2, dotprod68/2, dotprod67/2, dotprod66/2, dotprod65/2, dotprod64/2, dotprod63/2, dotprod62/2, dotprod61/2, dotprod60/2, dotprod59/2, dotprod58/2, dotprod57/2, dotprod56/2, dotprod55/2, dotprod54/2, dotprod53/2, dotprod52/2, dotprod51/2, dotprod50/2, dotprod49/2, dotprod48/2, dotprod47/2, dotprod46/2, dotprod45/2, dotprod44/2, dotprod43/2, dotprod42/2, dotprod41/2, dotprod40/2, dotprod39/2, dotprod38/2, dotprod37/2, dotprod36/2, dotprod35/2, dotprod34/2, dotprod33/2, dotprod32/2, dotprod31/2, dotprod30/2, dotprod29/2, dotprod28/2, dotprod27/2, dotprod26/2, dotprod25/2, dotprod24/2, dotprod23/2, dotprod22/2, dotprod21/2, dotprod20/2, dotprod19/2, dotprod18/2, dotprod17/2, dotprod16/2, dotprod15/2, dotprod14/2, dotprod13/2, dotprod12/2, dotprod11/2, dotprod10/2, dotprod9/2, dotprod8/2, dotprod7/2, dotprod6/2, dotprod5/2, dotprod4/2, dotprod3/2, dotprod2/2, dotprod1/2
  "IW{1,1}(1,:)'"/1 -> dotprod1/1
